simulink model "LCK_AVP"  (R2018b)
settings: Solver=FixedStepDiscrete  StartTime=0.0  StopTime=inf  FixedStep=0.01  RelTol=1e-3
PreLoadFcn:
  | if exist('tl_preloadfcn','file'), tl_preloadfcn(gcs,'4.4.0.41'); end
PostLoadFcn:
  | if any(exist('dsrtsu_mdlpostloadfcn', 'file') ~= 0), dsrtsu_mdlpostloadfcn('Execute', bdroot); end
  | if exist('tl_postloadfcn','file'), tl_postloadfcn(gcs,'4.4.0.41'); end
InitFcn:
  | if exist('tlds_init','file'), tlds_init(gcs); end
StartFcn:
  | if exist('tlds_start','file'), tlds_start(gcs); end
StopFcn:
  | if exist('tlds_stop','file'), tlds_stop(gcs); end
values from neighbouring files (symbols this model uses):
  C_DEG2RAD = 0.0175    [LCK_Macro.sldd]
  C_KPH2MPS = 0.2778    [LCK_Macro.sldd]
  C_NEARZERO = 0.0001    [LCK_Macro.sldd]
  C_ONE = 1.0    [LCK_Macro.sldd]
  C_RAD2DEG = 57.2958    [LCK_Macro.sldd]
  C_ZERO = 0.0    [LCK_Macro.sldd]
  k_accel_pedal_pos_per_speed_x : value not decoded    [LCK_LogicPara.sldd]
  k_accel_pedal_pos_per_speed_z : value not decoded    [LCK_LogicPara.sldd]
  k_brake_suprress_hold = 1000.0    [LCK_LogicPara.sldd]
  k_driver_appl_torque_filt = 50.0    [LCK_LogicPara.sldd]
  k_driver_suppression_hold_time = 3000.0    [LCK_LogicPara.sldd]
  k_hands_on_wheel_hold_msec = 500.0    [LCK_LogicPara.sldd]
  k_hands_on_wheel_torque_hi = 0.2    [LCK_LogicPara.sldd]
  k_hands_on_wheel_torque_lo = 0.15    [LCK_LogicPara.sldd]
  k_handsoff_delay_cycles = 50.0    [LCK_LogicPara.sldd]
  k_handsoff_torq_Lo_CR = 0.3    [LCK_LogicPara.sldd]
  k_handson_delay_cycles = 5.0    [LCK_LogicPara.sldd]
  k_HighAccel_suppress_hold = 3000.0    [LCK_LogicPara.sldd]
  k_HLR_suprress_hold = 3000.0    [LCK_LogicPara.sldd]
  k_hs_StrAng_CR_threshold_z : value not decoded    [LCK_LogicPara.sldd]
  k_LC_Exit_Switch = 0.0    [LCK_LogicPara.sldd]
  k_LCG_Configured = 1.0    [LCK_LogicPara.sldd]
  k_LCK_A0_Rdy2Act_UseConst = 0.0    [LCK_LogicPara.sldd]
  k_LCK_A0Fac_ActSta : value not decoded    [LCK_CtrlPara.sldd]
  k_LCK_A0Fac_DrvStm : value not decoded    [LCK_CtrlPara.sldd]
  k_LCK_A0Shift_LftCurv : value not decoded    [LCK_CtrlPara.sldd]
  k_LCK_A0Shift_RgtCurv : value not decoded    [LCK_CtrlPara.sldd]
  k_LCK_A0Shift_StraLan = 0.0    [LCK_CtrlPara.sldd]
  k_LCK_A0ShiftFac_Dy_LftCurv : value not decoded    [LCK_CtrlPara.sldd]
  k_LCK_A0ShiftFac_Dy_RgtCurv : value not decoded    [LCK_CtrlPara.sldd]
  k_LCK_A0ShiftFac_Vspd : value not decoded    [LCK_CtrlPara.sldd]
  k_LCK_accel_inhibit_thold = 35.0    [LCK_LogicPara.sldd]
  k_LCK_Active2Ready_Mask = 255.0    [LCK_LogicPara.sldd]
  k_LCK_CvatRateBks : value not decoded    [LCK_CtrlPara.sldd]
  k_LCK_CvatrBks : value not decoded    [LCK_CtrlPara.sldd]
  k_LCK_DFac_Dy : value not decoded    [LCK_CtrlPara.sldd]
  k_LCK_DFac_Dy_Curv : value not decoded    [LCK_CtrlPara.sldd]
  k_LCK_DFac_HaCurCen : value not decoded    [LCK_CtrlPara.sldd]
  k_LCK_DFac_HaCurSid : value not decoded    [LCK_CtrlPara.sldd]
  k_LCK_DFac_HadCurCen : value not decoded    [LCK_CtrlPara.sldd]
  k_LCK_DFac_HadCurSid : value not decoded    [LCK_CtrlPara.sldd]
  k_LCK_DFac_HadStrCen : value not decoded    [LCK_CtrlPara.sldd]
  k_LCK_DFac_HadStrSid : value not decoded    [LCK_CtrlPara.sldd]
  k_LCK_DFac_HaStrCen : value not decoded    [LCK_CtrlPara.sldd]
  k_LCK_DFac_HaStrSid : value not decoded    [LCK_CtrlPara.sldd]
  k_LCK_DFac_Rad : value not decoded    [LCK_CtrlPara.sldd]
  k_LCK_DFac_SA_CurCen : value not decoded    [LCK_CtrlPara.sldd]
  k_LCK_DFac_SA_CurSid : value not decoded    [LCK_CtrlPara.sldd]
  k_LCK_DFac_SA_StrCen : value not decoded    [LCK_CtrlPara.sldd]
  k_LCK_DFac_SA_StrSid : value not decoded    [LCK_CtrlPara.sldd]
  k_LCK_DFac_SS_CurCen : value not decoded    [LCK_CtrlPara.sldd]
  k_LCK_DFac_SS_CurSid : value not decoded    [LCK_CtrlPara.sldd]
  k_LCK_DFac_SS_StrCen : value not decoded    [LCK_CtrlPara.sldd]
  k_LCK_DFac_SS_StrSid : value not decoded    [LCK_CtrlPara.sldd]
  k_LCK_DFac_Vspd : value not decoded    [LCK_CtrlPara.sldd]
  k_LCK_DlyTm_DrvStim = 0.2    [LCK_CtrlPara.sldd]
  k_LCK_DTermMax = 2.0    [LCK_CtrlPara.sldd]
  k_LCK_DyBks_Curv : value not decoded    [LCK_CtrlPara.sldd]
  k_LCK_Enable_POOnly = 1.0    [LCK_LogicPara.sldd]
  k_LCK_Entry_DistBuffer = 0.1    [LCK_LogicPara.sldd]
  k_LCK_Fac_Vspd2RngThr_FalRec = 0.23    [LCK_CtrlPara.sldd]
  k_LCK_Ffw_CvatSwh = 0.0    [LCK_CtrlPara.sldd]
  k_LCK_Ffw_DyBks : value not decoded    [LCK_CtrlPara.sldd]
  k_LCK_Ffw_TimCon_CmdFlt = 0.0    [LCK_CtrlPara.sldd]
  k_LCK_FfwDeltaFac_Rad_Lft : value not decoded    [LCK_CtrlPara.sldd]
  k_LCK_FfwDeltaFac_Rad_Rgt : value not decoded    [LCK_CtrlPara.sldd]
  k_LCK_FfwDeltaFac_Vspd : value not decoded    [LCK_CtrlPara.sldd]
  k_LCK_FfwFac_CvatRate_Lft : value not decoded    [LCK_CtrlPara.sldd]
  k_LCK_FfwFac_CvatRate_Rgt : value not decoded    [LCK_CtrlPara.sldd]
  k_LCK_FfwFac_Dy : value not decoded    [LCK_CtrlPara.sldd]
  k_LCK_FfwFac_Rad_Lft : value not decoded    [LCK_CtrlPara.sldd]
  k_LCK_FfwFac_Rad_Rgt : value not decoded    [LCK_CtrlPara.sldd]
  k_LCK_FfwFac_Vspd : value not decoded    [LCK_CtrlPara.sldd]
  k_LCK_FfwTorq_Cvat : value not decoded    [LCK_CtrlPara.sldd]
  k_LCK_HAFac_ActSta : value not decoded    [LCK_CtrlPara.sldd]
  k_LCK_HAFac_DrvStm : value not decoded    [LCK_CtrlPara.sldd]
  k_LCK_HaloTime = 2000.0    [LCK_LogicPara.sldd]
  k_LCK_HaloTime_Switch = 0.0    [LCK_LogicPara.sldd]
  k_LCK_HARFac_ActSta : value not decoded    [LCK_CtrlPara.sldd]
  k_LCK_HARFac_DrvStm : value not decoded    [LCK_CtrlPara.sldd]
  k_LCK_Hed_DyBks : value not decoded    [LCK_CtrlPara.sldd]
  k_LCK_HedAngDiffX : value not decoded    [LCK_CtrlPara.sldd]
  k_LCK_HedAngRateDiffX : value not decoded    [LCK_CtrlPara.sldd]
  k_LCK_HndsOnWhel_DlyTm_Idl2Rdy = 0.0    [LCK_LogicPara.sldd]
  k_LCK_host_veh_width = 1.86    [LCK_LogicPara.sldd]
  k_LCK_Idle2Ready_Mask = 239.0    [LCK_LogicPara.sldd]
  k_LCK_Junc_SusTime = 1.0    [LCK_LogicPara.sldd]
  k_LCK_KpKdDecSlopeLmt = 10.0    [LCK_CtrlPara.sldd]
  k_LCK_KpKdIncSlopeLmt = 5.0    [LCK_CtrlPara.sldd]
  k_LCK_Lat_Ctrl_DFac_Lft = 1.0    [LCK_CtrlPara.sldd]
  k_LCK_Lat_Ctrl_DFac_Rgt = 1.05    [LCK_CtrlPara.sldd]
  k_LCK_Lat_Ctrl_Kd = 0.8    [LCK_CtrlPara.sldd]
  k_LCK_Lat_Ctrl_Ki = 0.5    [LCK_CtrlPara.sldd]
  k_LCK_Lat_Ctrl_Kp = 0.7    [LCK_CtrlPara.sldd]
  k_LCK_Lat_Ctrl_Kp_NearGain = 0.7    [LCK_CtrlPara.sldd]
  k_LCK_Lat_Ctrl_PFac_Lft = 1.0    [LCK_CtrlPara.sldd]
  k_LCK_Lat_Ctrl_PFac_Rgt = 1.05    [LCK_CtrlPara.sldd]
  k_LCK_Lat_Ctrl_TimCon_CmdFlt = 5.0    [LCK_CtrlPara.sldd]
  k_LCK_Lat_DFac_Rad : value not decoded    [LCK_CtrlPara.sldd]
  k_LCK_Lat_DFac_SS_Cur : value not decoded    [LCK_CtrlPara.sldd]
  k_LCK_Lat_DFac_SS_Str : value not decoded    [LCK_CtrlPara.sldd]
  k_LCK_Lat_DFac_Vspd : value not decoded    [LCK_CtrlPara.sldd]
  k_LCK_Lat_DyBks : value not decoded    [LCK_CtrlPara.sldd]
  k_LCK_Lat_IFac_Rad : value not decoded    [LCK_CtrlPara.sldd]
  k_LCK_Lat_IFac_Vspd : value not decoded    [LCK_CtrlPara.sldd]
  k_LCK_Lat_ILmtFac_Dy_CurvLan : value not decoded    [LCK_CtrlPara.sldd]
  k_LCK_Lat_ILmtFac_Dy_StraLan : value not decoded    [LCK_CtrlPara.sldd]
  k_LCK_Lat_ILmtFac_Rad : value not decoded    [LCK_CtrlPara.sldd]
  k_LCK_Lat_ILmtFac_Rad_NearGain = 1.0    [LCK_CtrlPara.sldd]
  k_LCK_Lat_ILmtFac_Vspd_CurvLan : value not decoded    [LCK_CtrlPara.sldd]
  k_LCK_Lat_ILmtFac_Vspd_StraLan : value not decoded    [LCK_CtrlPara.sldd]
  k_LCK_Lat_ITermLmt_Dy = 1.0    [LCK_CtrlPara.sldd]
  k_LCK_Lat_KpKdDecSlopeLmt = 10.0    [LCK_CtrlPara.sldd]
  k_LCK_Lat_KpKdIncSlopeLmt = 10.0    [LCK_CtrlPara.sldd]
  k_LCK_Lat_PFac_Dy_InnLftCur : value not decoded    [LCK_CtrlPara.sldd]
  k_LCK_Lat_PFac_Dy_InnRgtCur : value not decoded    [LCK_CtrlPara.sldd]
  k_LCK_Lat_PFac_Dy_OutLftCur : value not decoded    [LCK_CtrlPara.sldd]
  k_LCK_Lat_PFac_Dy_OutRgtCur : value not decoded    [LCK_CtrlPara.sldd]
  k_LCK_Lat_PFac_Dy_Str : value not decoded    [LCK_CtrlPara.sldd]
  k_LCK_Lat_PFac_Rad : value not decoded    [LCK_CtrlPara.sldd]
  ... (+153 more)
undefined symbols (not defined in the file or in its folder): k_LCK_CurvBks, K_LCK_SPA0A1A2_LMRngCmp_y
libraries: LateralControl_fcns_lib x58, simulink x24
(part 42 of 48)

== system LCK_AVP/Lateral_Control_Module/Adas_Lateral_Control_LCK_Core/Module 9/Module 0/Definition Fac 2 ==
  Hed_Ang : Inport
  Cen_Flag : Inport  Port=2
  Str_Flag : Inport  Port=3
  Abs2 : Abs
  Switch{1..4,9..10} (6 alike) : Switch  Criteria=u2 > Threshold
  k_LCK_DFac_HaCurCen : Lookup_n-D  NumberOfTableDimensions=1  BreakpointsForDimension1=k_LCK_HedAngDiffX  IndexSearchMethod=Linear search  Table=k_LCK_DFac_HaCurCen  ExtrapMethod=Clip  InternalRulePriority=Speed  RndMeth=Simplest  InputSameDT=on
  k_LCK_DFac_HaCurSid : Lookup_n-D  NumberOfTableDimensions=1  BreakpointsForDimension1=k_LCK_HedAngDiffX  IndexSearchMethod=Linear search  Table=k_LCK_DFac_HaCurSid  ExtrapMethod=Clip  InternalRulePriority=Speed  RndMeth=Simplest  InputSameDT=on
  k_LCK_DFac_HaStrCen : Lookup_n-D  NumberOfTableDimensions=1  BreakpointsForDimension1=k_LCK_HedAngDiffX  IndexSearchMethod=Linear search  Table=k_LCK_DFac_HaStrCen  ExtrapMethod=Clip  InternalRulePriority=Speed  RndMeth=Simplest  InputSameDT=on
  k_LCK_DFac_HaStrSid : Lookup_n-D  NumberOfTableDimensions=1  BreakpointsForDimension1=k_LCK_HedAngDiffX  IndexSearchMethod=Linear search  Table=k_LCK_DFac_HaStrSid  ExtrapMethod=Clip  InternalRulePriority=Speed  RndMeth=Simplest  InputSameDT=on
  k_LCK_PFac_HaCurCen : Lookup_n-D  NumberOfTableDimensions=1  BreakpointsForDimension1=k_LCK_HedAngDiffX  IndexSearchMethod=Linear search  Table=k_LCK_PFac_HaCurCen  ExtrapMethod=Clip  InternalRulePriority=Speed  RndMeth=Simplest  InputSameDT=on
  k_LCK_PFac_HaCurSid : Lookup_n-D  NumberOfTableDimensions=1  BreakpointsForDimension1=k_LCK_HedAngDiffX  IndexSearchMethod=Linear search  Table=k_LCK_PFac_HaCurSid  ExtrapMethod=Clip  InternalRulePriority=Speed  RndMeth=Simplest  InputSameDT=on
  k_LCK_PFac_HaStrSid : Lookup_n-D  NumberOfTableDimensions=1  BreakpointsForDimension1=k_LCK_HedAngDiffX  IndexSearchMethod=Linear search  Table=k_LCK_PFac_HaStrSid  ExtrapMethod=Clip  InternalRulePriority=Speed  RndMeth=Simplest  InputSameDT=on
  k_LCK_PFac_Ha_StrCen : Lookup_n-D  NumberOfTableDimensions=1  BreakpointsForDimension1=k_LCK_HedAngDiffX  IndexSearchMethod=Linear search  Table=k_LCK_PFac_HaStrCen  ExtrapMethod=Clip  InternalRulePriority=Speed  RndMeth=Simplest  InputSameDT=on
  LatCtrl_PFac_HedAngDiff : Outport
  LatCtrl_DFac_HedAngDiff : Outport  Port=2
  wires:
  k_LCK_PFac_HaCurSid/1 -> Switch3/3
  k_LCK_DFac_HaStrCen/1 -> Switch2/1
  k_LCK_DFac_HaCurSid/1 -> Switch4/3
  Abs2/1 -> k_LCK_PFac_HaStrSid/1, k_LCK_DFac_HaCurSid/1, k_LCK_DFac_HaCurCen/1, k_LCK_DFac_HaStrSid/1, k_LCK_DFac_HaStrCen/1, k_LCK_PFac_HaCurSid/1, k_LCK_PFac_HaCurCen/1, k_LCK_PFac_Ha_StrCen/1
  k_LCK_PFac_HaCurCen/1 -> Switch3/1
  k_LCK_DFac_HaCurCen/1 -> Switch4/1
  k_LCK_PFac_HaStrSid/1 -> Switch1/3
  k_LCK_PFac_Ha_StrCen/1 -> Switch1/1
  k_LCK_DFac_HaStrSid/1 -> Switch2/3
  Hed_Ang/1 -> Abs2/1
  Cen_Flag/1 -> Switch2/2, Switch4/2, Switch3/2, Switch1/2
  Switch3/1 -> Switch9/3
  Switch1/1 -> Switch9/1
  Switch10/1 -> LatCtrl_DFac_HedAngDiff/1
  Switch9/1 -> LatCtrl_PFac_HedAngDiff/1
  Switch2/1 -> Switch10/1
  Str_Flag/1 -> Switch9/2, Switch10/2
  Switch4/1 -> Switch10/3

== system LCK_AVP/Lateral_Control_Module/Adas_Lateral_Control_LCK_Core/Module 9/Module 0/Definition Fac 3 ==
  Hed_Ang_Diff_Rat : Inport
  Cen_Flag : Inport  Port=2
  Str_Flag : Inport  Port=3
  Abs3 : Abs
  Switch{5..8,11..12} (6 alike) : Switch  Criteria=u2 > Threshold
  k_LCK_DFac_HadCurCen : Lookup_n-D  NumberOfTableDimensions=1  BreakpointsForDimension1=k_LCK_HedAngRateDiffX  IndexSearchMethod=Linear search  Table=k_LCK_DFac_HadCurCen  ExtrapMethod=Clip  InternalRulePriority=Speed  RndMeth=Simplest  InputSameDT=on
  k_LCK_DFac_HadCurSid : Lookup_n-D  NumberOfTableDimensions=1  BreakpointsForDimension1=k_LCK_HedAngRateDiffX  IndexSearchMethod=Linear search  Table=k_LCK_DFac_HadCurSid  ExtrapMethod=Clip  InternalRulePriority=Speed  RndMeth=Simplest  InputSameDT=on
  k_LCK_DFac_HadStrCen : Lookup_n-D  NumberOfTableDimensions=1  BreakpointsForDimension1=k_LCK_HedAngRateDiffX  IndexSearchMethod=Linear search  Table=k_LCK_DFac_HadStrCen  ExtrapMethod=Clip  InternalRulePriority=Speed  RndMeth=Simplest  InputSameDT=on
  k_LCK_DFac_HadStrSid : Lookup_n-D  NumberOfTableDimensions=1  BreakpointsForDimension1=k_LCK_HedAngRateDiffX  IndexSearchMethod=Linear search  Table=k_LCK_DFac_HadStrSid  ExtrapMethod=Clip  InternalRulePriority=Speed  RndMeth=Simplest  InputSameDT=on
  k_LCK_PFac_HadCurCen : Lookup_n-D  NumberOfTableDimensions=1  BreakpointsForDimension1=k_LCK_HedAngRateDiffX  IndexSearchMethod=Linear search  Table=k_LCK_PFac_HadCurCen  ExtrapMethod=Clip  InternalRulePriority=Speed  RndMeth=Simplest  InputSameDT=on
  k_LCK_PFac_HadCurSid : Lookup_n-D  NumberOfTableDimensions=1  BreakpointsForDimension1=k_LCK_HedAngRateDiffX  IndexSearchMethod=Linear search  Table=k_LCK_PFac_HadCurSid  ExtrapMethod=Clip  InternalRulePriority=Speed  RndMeth=Simplest  InputSameDT=on
  k_LCK_PFac_HadStrCen : Lookup_n-D  NumberOfTableDimensions=1  BreakpointsForDimension1=k_LCK_HedAngRateDiffX  IndexSearchMethod=Linear search  Table=k_LCK_PFac_HadStrCen  ExtrapMethod=Clip  InternalRulePriority=Speed  RndMeth=Simplest  InputSameDT=on
  k_LCK_PFac_HadStrSid : Lookup_n-D  NumberOfTableDimensions=1  BreakpointsForDimension1=k_LCK_HedAngRateDiffX  IndexSearchMethod=Linear search  Table=k_LCK_PFac_HadStrSid  ExtrapMethod=Clip  InternalRulePriority=Speed  RndMeth=Simplest  InputSameDT=on
  LatCtrl_PFac_HedAngDiffRat : Outport
  LatCtrl_DFac_HedAngDiffRat : Outport  Port=2
  wires:
  Abs3/1 -> k_LCK_PFac_HadStrCen/1, k_LCK_PFac_HadCurSid/1, k_LCK_DFac_HadCurSid/1, k_LCK_DFac_HadCurCen/1, k_LCK_DFac_HadStrSid/1, k_LCK_DFac_HadStrCen/1, k_LCK_PFac_HadCurCen/1, k_LCK_PFac_HadStrSid/1
  k_LCK_DFac_HadStrCen/1 -> Switch7/1
  k_LCK_DFac_HadStrSid/1 -> Switch7/3
  k_LCK_PFac_HadCurSid/1 -> Switch6/3
  k_LCK_PFac_HadCurCen/1 -> Switch6/1
  Hed_Ang_Diff_Rat/1 -> Abs3/1
  Cen_Flag/1 -> Switch8/2, Switch7/2, Switch6/2, Switch5/2
  k_LCK_DFac_HadCurSid/1 -> Switch8/3
  k_LCK_DFac_HadCurCen/1 -> Switch8/1
  Switch12/1 -> LatCtrl_PFac_HedAngDiffRat/1
  Switch11/1 -> LatCtrl_DFac_HedAngDiffRat/1
  Switch5/1 -> Switch12/1
  Switch7/1 -> Switch11/1
  Switch8/1 -> Switch11/3
  Switch6/1 -> Switch12/3
  Str_Flag/1 -> Switch11/2, Switch12/2
  k_LCK_PFac_HadStrSid/1 -> Switch5/3
  k_LCK_PFac_HadStrCen/1 -> Switch5/1
